simulink model "simulation"  (R2015a)
settings: Solver=ode45  StartTime=0.0  StopTime=10.0  RelTol=1e-3
values from neighbouring files (symbols this model uses):
  mu = 5    [main - Kopi.m]    (also in main.m; main_2.m; oving_0.mat)
  x1_0 = 5    [main - Kopi.m]    (also in main.m = 1; main_2.m = x1_0_verdier(i); oving_0.mat = 2)
  x2_0 = 5    [main - Kopi.m]    (also in main.m = 1; main_2.m = x2_0_verdier(i); oving_0.mat = -1)
settings Model: Creator=RenCale  LastModifiedBy=RenCale

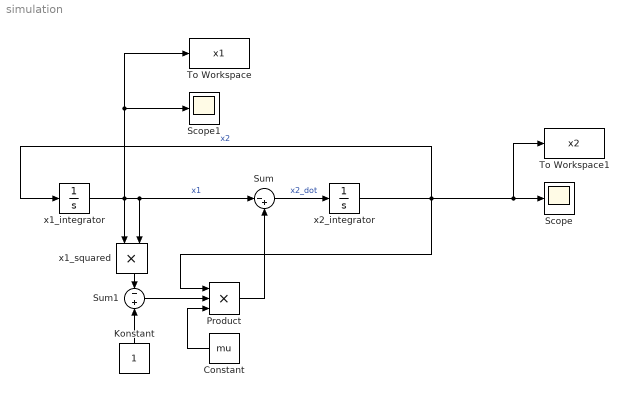
== system simulation ==
  Constant : Constant  Value=mu
  Konstant : Constant
  Product : Product  Inputs=3
  Scope : Scope
  Scope1 : Scope
  Sum : Sum  Inputs=|-+
  Sum1 : Sum  Inputs=-|+
  To Workspace : ToWorkspace  VariableName=x1  SaveFormat=Timeseries  SampleTime=-1
  To Workspace1 : ToWorkspace  VariableName=x2  SaveFormat=Timeseries  SampleTime=-1
  x1_integrator : Integrator  InitialCondition=x1_0
  x1_squared : Product
  x2_integrator : Integrator  InitialCondition=x2_0
  wires:
  x2_integrator/1 -> x1_integrator/1, To Workspace1/1, Scope/1, Product/1  "x2"
  Sum/1 -> x2_integrator/1  "x2_dot"
  x1_integrator/1 -> To Workspace/1, Scope1/1, x1_squared/1, Sum/1, x1_squared/2  "x1"
  x1_squared/1 -> Sum1/1
  Konstant/1 -> Sum1/2
  Sum1/1 -> Product/2
  Constant/1 -> Product/3
  Product/1 -> Sum/2
